simulink model "simoct21"  (R2023b)
settings: Solver=VariableStepAuto  StartTime=0.0  StopTime=10.0  RelTol=1e-3
settings Model: Creator=20808  LastModifiedBy=20808

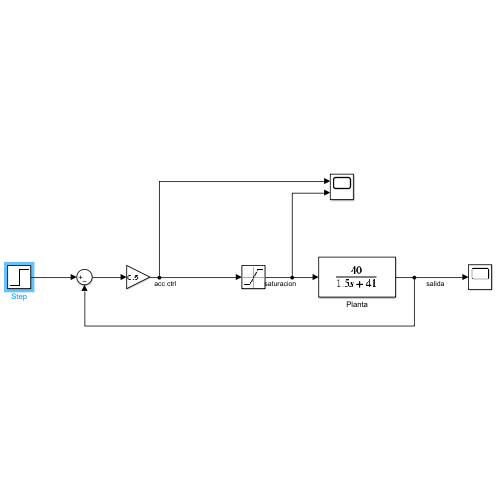
[thumbnail: Simulink's stored preview of the top-level diagram]
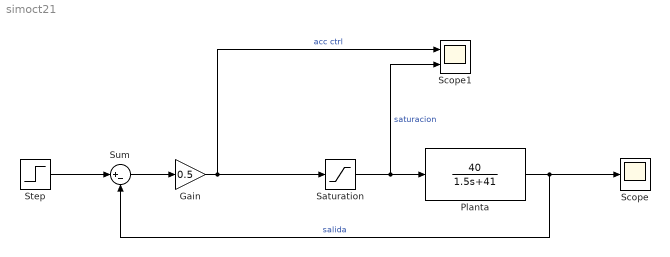
== system simoct21 ==
  Gain : Gain  Gain=0.5
  Planta : TransferFcn  Numerator=[40]  Denominator=[1.5 41]
  Saturation : Saturate
  Scope : Scope
  Scope1 : Scope  NumInputPorts=2
  Step : Step  After=0.1  SampleTime=0
  Sum : Sum  Inputs=|+-
  wires:
  Step/1 -> Sum/1
  Sum/1 -> Gain/1
  Gain/1 -> Saturation/1, Scope1/1  "acc ctrl"
  Planta/1 -> Scope/1, Sum/2  "salida"
  Saturation/1 -> Planta/1, Scope1/2  "saturacion"
